simulink model "main_PETC"  (R2021a)
settings: Solver=VariableStepAuto  StartTime=0.0  StopTime=10  FixedStep=1e-4  RelTol=1e-3
InitFcn:
  | run('Parameter.m')
values from neighbouring files (symbols this model uses):
  cp = 1    [Parameter.m]
  cv = 5    [Parameter.m]
  cw = 5    [Parameter.m]
  fref = 60    [Parameter.m]
  Lc1 = 0.35e-3    (= 0.00035)    [Parameter.m]
  Lc2 = 0.35e-3    (= 0.00035)    [Parameter.m]
  Lc3 = 0.35e-3    (= 0.00035)    [Parameter.m]
  Lc4 = 0.35e-3    (= 0.00035)    [Parameter.m]
  Lt12 = 318e-6    (= 0.000318)    [Parameter.m]
  Lt23 = 1847e-6    (= 0.001847)    [Parameter.m]
  Lt34 = 318e-6    (= 0.000318)    [Parameter.m]
  Mp1 = 9.4e-5    (= 9.4e-05)    [Parameter.m]
  Mp2 = 9.4e-5    (= 9.4e-05)    [Parameter.m]
  Mp3 = 12.5e-5    (= 0.000125)    [Parameter.m]
  Mp4 = 12.5e-5    (= 0.000125)    [Parameter.m]
  Nq1 = 1.3e-3    (= 0.0013)    [Parameter.m]
  Nq2 = 1.3e-3    (= 0.0013)    [Parameter.m]
  Nq3 = 1.5e-3    (= 0.0015)    [Parameter.m]
  Nq4 = 1.5e-3    (= 0.0015)    [Parameter.m]
  Rc1 = 0.03    [Parameter.m]
  Rc2 = 0.03    [Parameter.m]
  Rc3 = 0.03    [Parameter.m]
  Rc4 = 0.03    [Parameter.m]
  Rt12 = 0.23    [Parameter.m]
  Rt23 = 0.35    [Parameter.m]
  Rt34 = 0.23    [Parameter.m]
  t2 = 1    [Parameter.m]    (also in wvpq_PETC.m)
  t3 = 10    [Parameter.m]
  t4 = 20    [Parameter.m]    (also in wvpq_PETC.m = 21)
  t5 = 35    [Parameter.m]    (also in wvpq_PETC.m = 33)
  t6 = 40    [Parameter.m]    (also in wvpq_PETC.m = 35)
  Uo = 220*sqrt(2)    [Parameter.m]
  vref = 380    [Parameter.m]
  wc = 31.4    [Parameter.m]
  wref = 2*pi*fref    (= 376.991118431)    [Parameter.m]
undefined symbols (not defined in the file or in its folder): gcbh, sps_rtmsupport
libraries: spsControlledVoltageSourceLib x12, spsAlphaBetaZerotodq0Lib x12, eeGeneralControl x8, spsThreePhaseSeriesRLCBranchLib x7, spsGroundLib x4, spsThreePhaseVIMeasurementLib x4, spsThreePhaseBreakerLib x4, spsPLL3phLib x4, spsThreePhaseSeriesRLCLoadLib x3, spspowerguiLib x1
(part 2 of 2)

== system main_PETC/controller 2/v_secondary 2 ==
  q2' : Inport
  Constant : Constant  Value=wc
  Gain1 : Gain  Gain=wc
  Gain11 : Gain  Gain=Nq2
  Gain5 : Gain  Gain=cv
  Integrator2 : Integrator  ExternalReset=rising
  Product : Product
  Step : Step  Time=t2  SampleTime=0
  Sum : Sum  Inputs=|+-
  Sum6 : Sum  Inputs=++|
  vn2 : Outport
  wires:
  [zv2] -> Gain5/1
  Sum/1 -> Gain11/1
  [q2] -> Gain1/1
  Gain11/1 -> Sum6/2
  Product/1 -> Sum/1
  q2'/1 -> Product/1
  Gain1/1 -> Sum/2
  Constant/1 -> Product/2
  Gain5/1 -> Sum6/1
  Sum6/1 -> Integrator2/1
  Step/1 -> Integrator2/2
  Integrator2/1 -> vn2/1

== system main_PETC/controller 2/w_secondary 2 ==
  Gain : Gain  Gain=cw
  Gain15 : Gain  Gain=cp
  Integrator : Integrator  ExternalReset=rising
  Step : Step  Time=t2  SampleTime=0
  Sum1 : Sum  Inputs=++|
  wn2 : Outport
  wires:
  [zp2] -> Gain15/1
  Integrator/1 -> wn2/1
  Gain15/1 -> Sum1/2
  [zw2] -> Gain/1
  Gain/1 -> Sum1/1
  Step/1 -> Integrator/2
  Sum1/1 -> Integrator/1

== system main_PETC/controller 3/(P) abc to dq2 ==
  abc : Inport  PortDimensions=3
  wt : Inport  Port=2  PortDimensions=1
  Alpha-Beta-Zero to dq0 : spsAlphaBetaZerotodq0Lib/Alpha-Beta-Zero to dq0  Alignment=90 degrees behind phase A axis
      settings: SourceProductBaseCode=PS
  abc to Alpha-Beta-Zero : Subsystem  AncestorBlock=powerlib_meascontrol/Transformations/abc to Alpha-Beta-Zero  DialogController=POWERSYS.PowerSysDialog  LoadFcn=sps_rtmsupport('LoadFcn', gcbh);  StartFcn=sps_rtmsupport('StartFcn', gcbh);  StopFcn=sps_rtmsupport('StopFcn', gcbh);  mask(abc to Alpha-Beta-Zero Transformation){}
      mask help: Perform a Clarke transformation from a three-phase (abc) signal to a alpha-beta-zero stationary reference frame.
      settings: CopyFcn=sps_rtmsupport('CopyFcn', gcbh);  DeleteFcn=sps_rtmsupport('DeleteFcn', gcbh);  UndoDeleteFcn=sps_rtmsupport('UndoDeleteFcn', gcbh);  ModelCloseFcn=sps_rtmsupport('ModelCloseFcn', gcbh);  PreSaveFcn=sps_rtmsupport('PreSaveFcn', gcbh);  PostSaveFcn=sps_rtmsupport('PostSaveFcn', gcbh);  NameChangeFcn=sps_rtmsupport('NameChangeFcn', gcbh);  PreCopyFcn=sps_rtmsupport('PreCopyFcn', gcbh);  OpenFcn=sps_rtmsupport('OpenFcn', gcbh, []);  CloseFcn=sps_rtmsupport('CloseFcn', gcbh);  PreDeleteFcn=sps_rtmsupport('PreDeleteFcn', gcbh);
      mask Help: helpview(psbhelp);
      mask Display:
      | plot([0 1], [0,1])
      | text(0.15,0.7,'abc')
      | text(0.55, 0.3,'\alpha\beta0','texmode','on')
  dq0 : Outport  VectorParamsAs1DForOutWhenUnconnected=off
  wires:
  wt/1 -> Alpha-Beta-Zero to dq0/2
  abc/1 -> abc to Alpha-Beta-Zero/1(abc)
  Alpha-Beta-Zero to dq0/1 -> dq0/1
  abc to Alpha-Beta-Zero/1(al_be_0) -> Alpha-Beta-Zero to dq0/1

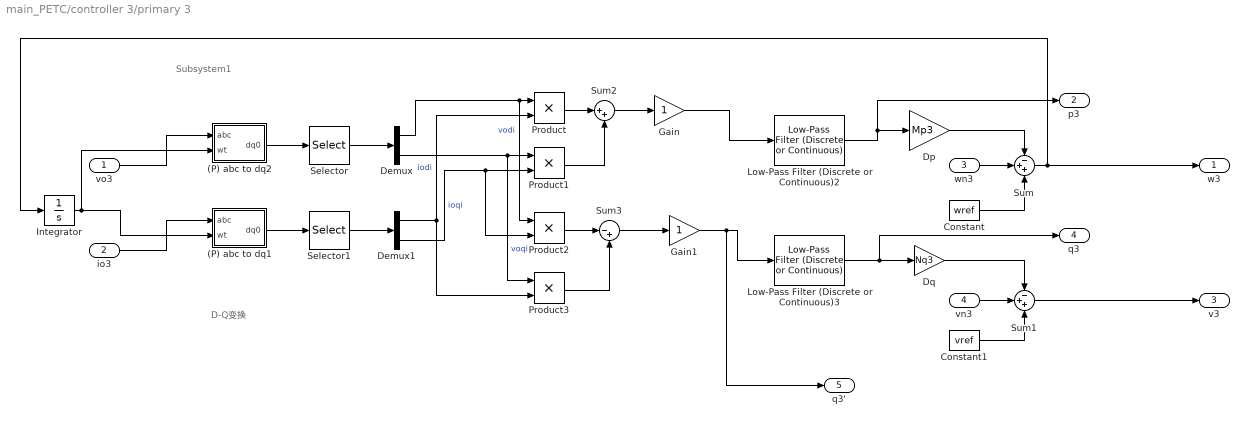
== system main_PETC/controller 3/primary 3 ==
  note: Subsystem1
  note: D-Q变换
  vo3 : Inport
  io3 : Inport  Port=2
  wn3 : Inport  Port=3
  vn3 : Inport  Port=4
  (P) abc to dq1 : Subsystem  AncestorBlock=powerlib_meascontrol/Transformations/abc to dq0  DialogController=POWERSYS.PowerSysDialog  LoadFcn=sps_rtmsupport('LoadFcn', gcbh);  StartFcn=sps_rtmsupport('StartFcn', gcbh);  StopFcn=sps_rtmsupport('StopFcn', gcbh);  mask(abc to dq0 Transformation){Alignment=90 degrees behind phase A axis}
      mask prompts: Alignment "Rotating frame alignment at wt=0:"
      mask help:
      | Perform a Park transformation from a three-phase (abc) signal to a dq0 rotating reference frame. Angular position of the rotating frame is given by input wt (rad).
      |
      | When the rotating frame alignment at wt=0 is 90 degrees behind phase A axis, a positive-sequence signal with Mag=1 & Phase=0 degrees yields the following dq values: d=1, q=0.
      mask init:
      | str=cat(2,gcb,'/Alpha-Beta-Zero to dq0');
      | if Alignment==1
      |     set_param(str,'Alignment','Aligned with phase A axis');
      | else
      |     set_param(str,'Alignment','90 degrees behind phase A axis');
      | end
      settings: CopyFcn=sps_rtmsupport('CopyFcn', gcbh);  DeleteFcn=sps_rtmsupport('DeleteFcn', gcbh);  UndoDeleteFcn=sps_rtmsupport('UndoDeleteFcn', gcbh);  ModelCloseFcn=sps_rtmsupport('ModelCloseFcn', gcbh);  PreSaveFcn=sps_rtmsupport('PreSaveFcn', gcbh);  PostSaveFcn=sps_rtmsupport('PostSaveFcn', gcbh);  NameChangeFcn=sps_rtmsupport('NameChangeFcn', gcbh);  PreCopyFcn=sps_rtmsupport('PreCopyFcn', gcbh);  OpenFcn=sps_rtmsupport('OpenFcn', gcbh, [1]);  CloseFcn=sps_rtmsupport('CloseFcn', gcbh);  PreDeleteFcn=sps_rtmsupport('PreDeleteFcn', gcbh);
      mask Help: helpview(psbhelp);
      mask TypeOptions Alignment: Aligned with phase A axis | 90 degrees behind phase A axis
      mask Display:
      | plot([0 1], [0,1])
      | port_label('input', 1, 'abc')
      | port_label('input', 2, 'wt')
      | port_label('output', 1, 'dq0')
  (P) abc to dq2 : Subsystem  AncestorBlock=powerlib_meascontrol/Transformations/abc to dq0  DialogController=POWERSYS.PowerSysDialog  LoadFcn=sps_rtmsupport('LoadFcn', gcbh);  StartFcn=sps_rtmsupport('StartFcn', gcbh);  StopFcn=sps_rtmsupport('StopFcn', gcbh);  mask(abc to dq0 Transformation){Alignment=90 degrees behind phase A axis}
      mask prompts: Alignment "Rotating frame alignment at wt=0:"
      mask help:
      | Perform a Park transformation from a three-phase (abc) signal to a dq0 rotating reference frame. Angular position of the rotating frame is given by input wt (rad).
      |
      | When the rotating frame alignment at wt=0 is 90 degrees behind phase A axis, a positive-sequence signal with Mag=1 & Phase=0 degrees yields the following dq values: d=1, q=0.
      mask init:
      | str=cat(2,gcb,'/Alpha-Beta-Zero to dq0');
      | if Alignment==1
      |     set_param(str,'Alignment','Aligned with phase A axis');
      | else
      |     set_param(str,'Alignment','90 degrees behind phase A axis');
      | end
      settings: CopyFcn=sps_rtmsupport('CopyFcn', gcbh);  DeleteFcn=sps_rtmsupport('DeleteFcn', gcbh);  UndoDeleteFcn=sps_rtmsupport('UndoDeleteFcn', gcbh);  ModelCloseFcn=sps_rtmsupport('ModelCloseFcn', gcbh);  PreSaveFcn=sps_rtmsupport('PreSaveFcn', gcbh);  PostSaveFcn=sps_rtmsupport('PostSaveFcn', gcbh);  NameChangeFcn=sps_rtmsupport('NameChangeFcn', gcbh);  PreCopyFcn=sps_rtmsupport('PreCopyFcn', gcbh);  OpenFcn=sps_rtmsupport('OpenFcn', gcbh, [1]);  CloseFcn=sps_rtmsupport('CloseFcn', gcbh);  PreDeleteFcn=sps_rtmsupport('PreDeleteFcn', gcbh);
      mask Help: helpview(psbhelp);
      mask TypeOptions Alignment: Aligned with phase A axis | 90 degrees behind phase A axis
      mask Display:
      | plot([0 1], [0,1])
      | port_label('input', 1, 'abc')
      | port_label('input', 2, 'wt')
      | port_label('output', 1, 'dq0')
  Constant : Constant  Value=wref
  Constant1 : Constant  Value=vref
  Demux : Demux  Outputs=2
  Demux1 : Demux  Outputs=2
  Dp : Gain  Gain=Mp3
  Dq : Gain  Gain=Nq3
  Gain : Gain
  Gain1 : Gain
  Integrator : Integrator
  Low-Pass Filter (Discrete or Continuous)2 : eeGeneralControl/Low-Pass Filter (Discrete or Continuous)  K=1  T=1/wc  B=inf  A=-inf  init_option=Inherited from block input  x0=0  Ts=-1
  Low-Pass Filter (Discrete or Continuous)3 : eeGeneralControl/Low-Pass Filter (Discrete or Continuous)  K=1  T=1/wc  B=inf  A=-inf  init_option=Inherited from block input  x0=0  Ts=-1
  Product{,1..3} (4 alike) : Product
  Selector : Selector  InputPortWidth=3  IndexOptions=Index vector (dialog)  Indices=[1 2]  OutputSizes=1
  Selector1 : Selector  InputPortWidth=3  IndexOptions=Index vector (dialog)  Indices=[1 2]  OutputSizes=1
  Sum : Sum  Inputs=-++
  Sum1 : Sum  Inputs=-++
  Sum2 : Sum  Inputs=|++
  Sum3 : Sum  Inputs=|-+
  w3 : Outport
  p3 : Outport  Port=2
  v3 : Outport  Port=3
  q3 : Outport  Port=4
  q3' : Outport  Port=5
  wires:
  vn3/1 -> Sum1/2
  Constant/1 -> Sum/3
  Sum1/1 -> v3/1
  Constant1/1 -> Sum1/3
  Low-Pass Filter (Discrete or Continuous)3/1 -> Dq/1, q3/1
  Sum/1 -> w3/1, Integrator/1
  Dq/1 -> Sum1/1
  wn3/1 -> Sum/2
  Dp/1 -> Sum/1
  Low-Pass Filter (Discrete or Continuous)2/1 -> Dp/1, p3/1
  Gain1/1 -> Low-Pass Filter (Discrete or Continuous)3/1, q3'/1
  Gain/1 -> Low-Pass Filter (Discrete or Continuous)2/1
  Sum3/1 -> Gain1/1
  Sum2/1 -> Gain/1
  vo3/1 -> (P) abc to dq2/1(abc)
  io3/1 -> (P) abc to dq1/1(abc)
  Product/1 -> Sum2/1
  Product1/1 -> Sum2/2
  Demux1/2 -> Product1/2, Product2/2  "ioqi"
  Product2/1 -> Sum3/1
  Product3/1 -> Sum3/2
  (P) abc to dq1/1(dq0) -> Selector1/1
  Demux1/1 -> Product3/2, Product/2  "iodi"
  (P) abc to dq2/1(dq0) -> Selector/1
  Demux/1 -> Product2/1, Product/1  "vodi"
  Integrator/1 -> (P) abc to dq1/2(wt), (P) abc to dq2/2(wt)
  Selector1/1 -> Demux1/1
  Demux/2 -> Product1/1, Product3/1  "voqi"
  Selector/1 -> Demux/1

== system main_PETC/controller 3/v_secondary 3 ==
  q3' : Inport
  Constant : Constant  Value=wc
  Gain1 : Gain  Gain=wc
  Gain11 : Gain  Gain=Nq3
  Gain5 : Gain  Gain=cv
  Integrator2 : Integrator  ExternalReset=rising
  Product : Product
  Subsystem2 : Subsystem
  Sum : Sum  Inputs=|+-
  Sum1 : Sum  Inputs=++|
  vn3 : Outport
  wires:
  [zv3] -> Gain5/1
  Gain5/1 -> Sum1/1
  Integrator2/1 -> vn3/1
  Gain11/1 -> Sum1/2
  Gain1/1 -> Sum/2
  Constant/1 -> Product/2
  q3'/1 -> Product/1
  [q3] -> Gain1/1
  Product/1 -> Sum/1
  Sum/1 -> Gain11/1
  [t] -> Integrator2/2
  Sum1/1 -> Subsystem2/1(In1)
  Subsystem2/1(Out1) -> Integrator2/1

== system main_PETC/controller 3/w_secondary 3 ==
  Gain1 : Gain  Gain=cw
  Gain15 : Gain  Gain=cp
  Integrator : Integrator  ExternalReset=rising
  Subsystem2 : Subsystem
  Sum6 : Sum  Inputs=++|
  wn3 : Outport
  wires:
  Integrator/1 -> wn3/1
  Gain15/1 -> Sum6/2
  [zw3] -> Gain1/1
  Gain1/1 -> Sum6/1
  [zp3] -> Gain15/1
  [t] -> Integrator/2
  Sum6/1 -> Subsystem2/1(In1)
  Subsystem2/1(Out1) -> Integrator/1

== system main_PETC/controller 4/(P) abc to dq2 ==
  abc : Inport  PortDimensions=3
  wt : Inport  Port=2  PortDimensions=1
  Alpha-Beta-Zero to dq0 : spsAlphaBetaZerotodq0Lib/Alpha-Beta-Zero to dq0  Alignment=90 degrees behind phase A axis
      settings: SourceProductBaseCode=PS
  abc to Alpha-Beta-Zero : Subsystem  AncestorBlock=powerlib_meascontrol/Transformations/abc to Alpha-Beta-Zero  DialogController=POWERSYS.PowerSysDialog  LoadFcn=sps_rtmsupport('LoadFcn', gcbh);  StartFcn=sps_rtmsupport('StartFcn', gcbh);  StopFcn=sps_rtmsupport('StopFcn', gcbh);  mask(abc to Alpha-Beta-Zero Transformation){}
      mask help: Perform a Clarke transformation from a three-phase (abc) signal to a alpha-beta-zero stationary reference frame.
      settings: CopyFcn=sps_rtmsupport('CopyFcn', gcbh);  DeleteFcn=sps_rtmsupport('DeleteFcn', gcbh);  UndoDeleteFcn=sps_rtmsupport('UndoDeleteFcn', gcbh);  ModelCloseFcn=sps_rtmsupport('ModelCloseFcn', gcbh);  PreSaveFcn=sps_rtmsupport('PreSaveFcn', gcbh);  PostSaveFcn=sps_rtmsupport('PostSaveFcn', gcbh);  NameChangeFcn=sps_rtmsupport('NameChangeFcn', gcbh);  PreCopyFcn=sps_rtmsupport('PreCopyFcn', gcbh);  OpenFcn=sps_rtmsupport('OpenFcn', gcbh, []);  CloseFcn=sps_rtmsupport('CloseFcn', gcbh);  PreDeleteFcn=sps_rtmsupport('PreDeleteFcn', gcbh);
      mask Help: helpview(psbhelp);
      mask Display:
      | plot([0 1], [0,1])
      | text(0.15,0.7,'abc')
      | text(0.55, 0.3,'\alpha\beta0','texmode','on')
  dq0 : Outport  VectorParamsAs1DForOutWhenUnconnected=off
  wires:
  wt/1 -> Alpha-Beta-Zero to dq0/2
  abc/1 -> abc to Alpha-Beta-Zero/1(abc)
  Alpha-Beta-Zero to dq0/1 -> dq0/1
  abc to Alpha-Beta-Zero/1(al_be_0) -> Alpha-Beta-Zero to dq0/1

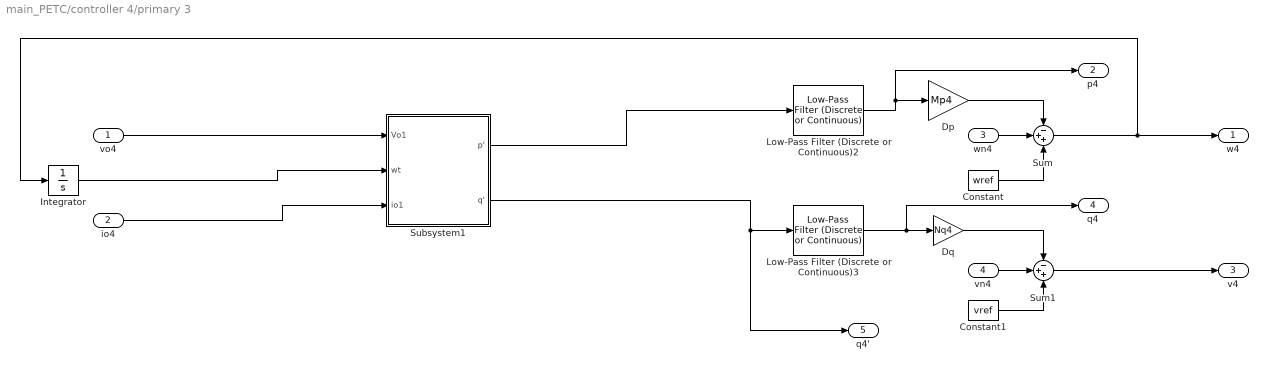
== system main_PETC/controller 4/primary 3 ==
  vo4 : Inport
  io4 : Inport  Port=2
  wn4 : Inport  Port=3
  vn4 : Inport  Port=4
  Constant : Constant  Value=wref
  Constant1 : Constant  Value=vref
  Dp : Gain  Gain=Mp4
  Dq : Gain  Gain=Nq4
  Integrator : Integrator
  Low-Pass Filter (Discrete or Continuous)2 : eeGeneralControl/Low-Pass Filter (Discrete or Continuous)  K=1  T=1/wc  B=inf  A=-inf  init_option=Inherited from block input  x0=0  Ts=-1
  Low-Pass Filter (Discrete or Continuous)3 : eeGeneralControl/Low-Pass Filter (Discrete or Continuous)  K=1  T=1/wc  B=inf  A=-inf  init_option=Inherited from block input  x0=0  Ts=-1
  Subsystem1 : Subsystem
  Sum : Sum  Inputs=-++
  Sum1 : Sum  Inputs=-++
  w4 : Outport
  p4 : Outport  Port=2
  v4 : Outport  Port=3
  q4 : Outport  Port=4
  q4' : Outport  Port=5
  wires:
  vn4/1 -> Sum1/2
  Constant/1 -> Sum/3
  Sum1/1 -> v4/1
  Constant1/1 -> Sum1/3
  Low-Pass Filter (Discrete or Continuous)3/1 -> Dq/1, q4/1
  Sum/1 -> w4/1, Integrator/1
  Dq/1 -> Sum1/1
  wn4/1 -> Sum/2
  Dp/1 -> Sum/1
  Low-Pass Filter (Discrete or Continuous)2/1 -> Dp/1, p4/1
  Subsystem1/2(q') -> Low-Pass Filter (Discrete or Continuous)3/1, q4'/1
  vo4/1 -> Subsystem1/1(Vo1)
  Integrator/1 -> Subsystem1/2(wt)
  io4/1 -> Subsystem1/3(io1)
  Subsystem1/1(p') -> Low-Pass Filter (Discrete or Continuous)2/1

== system main_PETC/controller 4/v_secondary 4 ==
  q4' : Inport
  Constant : Constant  Value=wc
  Gain1 : Gain  Gain=wc
  Gain11 : Gain  Gain=Nq4
  Gain5 : Gain  Gain=cv
  Integrator2 : Integrator  ExternalReset=rising
  Product : Product
  Step : Step  Time=t2  SampleTime=0
  Sum : Sum  Inputs=|+-
  Sum6 : Sum  Inputs=++|
  vn4 : Outport
  wires:
  [zv4] -> Gain5/1
  Integrator2/1 -> vn4/1
  Gain11/1 -> Sum6/2
  Sum6/1 -> Integrator2/1
  Gain1/1 -> Sum/2
  Constant/1 -> Product/2
  q4'/1 -> Product/1
  [q4] -> Gain1/1
  Product/1 -> Sum/1
  Sum/1 -> Gain11/1
  Step/1 -> Integrator2/2
  Gain5/1 -> Sum6/1

== system main_PETC/controller 4/w_secondary 4 ==
  Gain1 : Gain  Gain=cw
  Gain15 : Gain  Gain=cp
  Integrator : Integrator  ExternalReset=rising
  Step : Step  Time=t2  SampleTime=0
  Sum6 : Sum  Inputs=++|
  wn4 : Outport
  wires:
  Integrator/1 -> wn4/1
  Sum6/1 -> Integrator/1
  Gain15/1 -> Sum6/2
  [zw4] -> Gain1/1
  Gain1/1 -> Sum6/1
  [zp4] -> Gain15/1
  Step/1 -> Integrator/2

== system main_PETC/controller 1/(P) abc to dq2/abc to Alpha-Beta-Zero ==
  abc : Inport  PortDimensions=3
  Gain1 : Gain  Gain=sqrt(2/3)  SaturateOnIntegerOverflow=on  OutDataTypeStr=Inherit: Same as input  ParamDataTypeStr=Inherit: Same as input
  Gain3 : Gain  Gain="[ 1   -1/2   -1/2; 0   sqrt(3)/2   -sqrt(3)/2; 1/sqrt(2)  1/sqrt(2)  1/sqrt(2) ]"  Multiplication=Matrix(K*u) (u vector)  SaturateOnIntegerOverflow=on  OutDataTypeStr=Inherit: Same as input  ParamDataTypeStr=Inherit: Same as input
  al_be_0 : Outport  VectorParamsAs1DForOutWhenUnconnected=off
  wires:
  abc/1 -> Gain3/1
  Gain3/1 -> Gain1/1
  Gain1/1 -> al_be_0/1

== system main_PETC/controller 1/primary 1/(P) abc to dq1 ==
  abc : Inport  PortDimensions=3
  wt : Inport  Port=2  PortDimensions=1
  Alpha-Beta-Zero to dq0 : spsAlphaBetaZerotodq0Lib/Alpha-Beta-Zero to dq0  Alignment=90 degrees behind phase A axis
      settings: SourceProductBaseCode=PS
  abc to Alpha-Beta-Zero : Subsystem  AncestorBlock=powerlib_meascontrol/Transformations/abc to Alpha-Beta-Zero  DialogController=POWERSYS.PowerSysDialog  LoadFcn=sps_rtmsupport('LoadFcn', gcbh);  StartFcn=sps_rtmsupport('StartFcn', gcbh);  StopFcn=sps_rtmsupport('StopFcn', gcbh);  mask(abc to Alpha-Beta-Zero Transformation){}
      mask help: Perform a Clarke transformation from a three-phase (abc) signal to a alpha-beta-zero stationary reference frame.
      settings: CopyFcn=sps_rtmsupport('CopyFcn', gcbh);  DeleteFcn=sps_rtmsupport('DeleteFcn', gcbh);  UndoDeleteFcn=sps_rtmsupport('UndoDeleteFcn', gcbh);  ModelCloseFcn=sps_rtmsupport('ModelCloseFcn', gcbh);  PreSaveFcn=sps_rtmsupport('PreSaveFcn', gcbh);  PostSaveFcn=sps_rtmsupport('PostSaveFcn', gcbh);  NameChangeFcn=sps_rtmsupport('NameChangeFcn', gcbh);  PreCopyFcn=sps_rtmsupport('PreCopyFcn', gcbh);  OpenFcn=sps_rtmsupport('OpenFcn', gcbh, []);  CloseFcn=sps_rtmsupport('CloseFcn', gcbh);  PreDeleteFcn=sps_rtmsupport('PreDeleteFcn', gcbh);
      mask Help: helpview(psbhelp);
      mask Display:
      | plot([0 1], [0,1])
      | text(0.15,0.7,'abc')
      | text(0.55, 0.3,'\alpha\beta0','texmode','on')
  dq0 : Outport  VectorParamsAs1DForOutWhenUnconnected=off
  wires:
  wt/1 -> Alpha-Beta-Zero to dq0/2
  abc/1 -> abc to Alpha-Beta-Zero/1(abc)
  Alpha-Beta-Zero to dq0/1 -> dq0/1
  abc to Alpha-Beta-Zero/1(al_be_0) -> Alpha-Beta-Zero to dq0/1

== system main_PETC/controller 1/primary 1/(P) abc to dq2 ==
  abc : Inport  PortDimensions=3
  wt : Inport  Port=2  PortDimensions=1
  Alpha-Beta-Zero to dq0 : spsAlphaBetaZerotodq0Lib/Alpha-Beta-Zero to dq0  Alignment=90 degrees behind phase A axis
      settings: SourceProductBaseCode=PS
  abc to Alpha-Beta-Zero : Subsystem  AncestorBlock=powerlib_meascontrol/Transformations/abc to Alpha-Beta-Zero  DialogController=POWERSYS.PowerSysDialog  LoadFcn=sps_rtmsupport('LoadFcn', gcbh);  StartFcn=sps_rtmsupport('StartFcn', gcbh);  StopFcn=sps_rtmsupport('StopFcn', gcbh);  mask(abc to Alpha-Beta-Zero Transformation){}
      mask help: Perform a Clarke transformation from a three-phase (abc) signal to a alpha-beta-zero stationary reference frame.
      settings: CopyFcn=sps_rtmsupport('CopyFcn', gcbh);  DeleteFcn=sps_rtmsupport('DeleteFcn', gcbh);  UndoDeleteFcn=sps_rtmsupport('UndoDeleteFcn', gcbh);  ModelCloseFcn=sps_rtmsupport('ModelCloseFcn', gcbh);  PreSaveFcn=sps_rtmsupport('PreSaveFcn', gcbh);  PostSaveFcn=sps_rtmsupport('PostSaveFcn', gcbh);  NameChangeFcn=sps_rtmsupport('NameChangeFcn', gcbh);  PreCopyFcn=sps_rtmsupport('PreCopyFcn', gcbh);  OpenFcn=sps_rtmsupport('OpenFcn', gcbh, []);  CloseFcn=sps_rtmsupport('CloseFcn', gcbh);  PreDeleteFcn=sps_rtmsupport('PreDeleteFcn', gcbh);
      mask Help: helpview(psbhelp);
      mask Display:
      | plot([0 1], [0,1])
      | text(0.15,0.7,'abc')
      | text(0.55, 0.3,'\alpha\beta0','texmode','on')
  dq0 : Outport  VectorParamsAs1DForOutWhenUnconnected=off
  wires:
  wt/1 -> Alpha-Beta-Zero to dq0/2
  abc/1 -> abc to Alpha-Beta-Zero/1(abc)
  Alpha-Beta-Zero to dq0/1 -> dq0/1
  abc to Alpha-Beta-Zero/1(al_be_0) -> Alpha-Beta-Zero to dq0/1

== system main_PETC/controller 2/(P) abc to dq2/abc to Alpha-Beta-Zero ==
  abc : Inport  PortDimensions=3
  Gain1 : Gain  Gain=sqrt(2/3)  SaturateOnIntegerOverflow=on  OutDataTypeStr=Inherit: Same as input  ParamDataTypeStr=Inherit: Same as input
  Gain3 : Gain  Gain="[ 1   -1/2   -1/2; 0   sqrt(3)/2   -sqrt(3)/2; 1/sqrt(2)  1/sqrt(2)  1/sqrt(2) ]"  Multiplication=Matrix(K*u) (u vector)  SaturateOnIntegerOverflow=on  OutDataTypeStr=Inherit: Same as input  ParamDataTypeStr=Inherit: Same as input
  al_be_0 : Outport  VectorParamsAs1DForOutWhenUnconnected=off
  wires:
  abc/1 -> Gain3/1
  Gain3/1 -> Gain1/1
  Gain1/1 -> al_be_0/1

== system main_PETC/controller 2/primary 1/(P) abc to dq1 ==
  abc : Inport  PortDimensions=3
  wt : Inport  Port=2  PortDimensions=1
  Alpha-Beta-Zero to dq0 : spsAlphaBetaZerotodq0Lib/Alpha-Beta-Zero to dq0  Alignment=90 degrees behind phase A axis
      settings: SourceProductBaseCode=PS
  abc to Alpha-Beta-Zero : Subsystem  AncestorBlock=powerlib_meascontrol/Transformations/abc to Alpha-Beta-Zero  DialogController=POWERSYS.PowerSysDialog  LoadFcn=sps_rtmsupport('LoadFcn', gcbh);  StartFcn=sps_rtmsupport('StartFcn', gcbh);  StopFcn=sps_rtmsupport('StopFcn', gcbh);  mask(abc to Alpha-Beta-Zero Transformation){}
      mask help: Perform a Clarke transformation from a three-phase (abc) signal to a alpha-beta-zero stationary reference frame.
      settings: CopyFcn=sps_rtmsupport('CopyFcn', gcbh);  DeleteFcn=sps_rtmsupport('DeleteFcn', gcbh);  UndoDeleteFcn=sps_rtmsupport('UndoDeleteFcn', gcbh);  ModelCloseFcn=sps_rtmsupport('ModelCloseFcn', gcbh);  PreSaveFcn=sps_rtmsupport('PreSaveFcn', gcbh);  PostSaveFcn=sps_rtmsupport('PostSaveFcn', gcbh);  NameChangeFcn=sps_rtmsupport('NameChangeFcn', gcbh);  PreCopyFcn=sps_rtmsupport('PreCopyFcn', gcbh);  OpenFcn=sps_rtmsupport('OpenFcn', gcbh, []);  CloseFcn=sps_rtmsupport('CloseFcn', gcbh);  PreDeleteFcn=sps_rtmsupport('PreDeleteFcn', gcbh);
      mask Help: helpview(psbhelp);
      mask Display:
      | plot([0 1], [0,1])
      | text(0.15,0.7,'abc')
      | text(0.55, 0.3,'\alpha\beta0','texmode','on')
  dq0 : Outport  VectorParamsAs1DForOutWhenUnconnected=off
  wires:
  wt/1 -> Alpha-Beta-Zero to dq0/2
  abc/1 -> abc to Alpha-Beta-Zero/1(abc)
  Alpha-Beta-Zero to dq0/1 -> dq0/1
  abc to Alpha-Beta-Zero/1(al_be_0) -> Alpha-Beta-Zero to dq0/1

== system main_PETC/controller 2/primary 1/(P) abc to dq2 ==
  abc : Inport  PortDimensions=3
  wt : Inport  Port=2  PortDimensions=1
  Alpha-Beta-Zero to dq0 : spsAlphaBetaZerotodq0Lib/Alpha-Beta-Zero to dq0  Alignment=90 degrees behind phase A axis
      settings: SourceProductBaseCode=PS
  abc to Alpha-Beta-Zero : Subsystem  AncestorBlock=powerlib_meascontrol/Transformations/abc to Alpha-Beta-Zero  DialogController=POWERSYS.PowerSysDialog  LoadFcn=sps_rtmsupport('LoadFcn', gcbh);  StartFcn=sps_rtmsupport('StartFcn', gcbh);  StopFcn=sps_rtmsupport('StopFcn', gcbh);  mask(abc to Alpha-Beta-Zero Transformation){}
      mask help: Perform a Clarke transformation from a three-phase (abc) signal to a alpha-beta-zero stationary reference frame.
      settings: CopyFcn=sps_rtmsupport('CopyFcn', gcbh);  DeleteFcn=sps_rtmsupport('DeleteFcn', gcbh);  UndoDeleteFcn=sps_rtmsupport('UndoDeleteFcn', gcbh);  ModelCloseFcn=sps_rtmsupport('ModelCloseFcn', gcbh);  PreSaveFcn=sps_rtmsupport('PreSaveFcn', gcbh);  PostSaveFcn=sps_rtmsupport('PostSaveFcn', gcbh);  NameChangeFcn=sps_rtmsupport('NameChangeFcn', gcbh);  PreCopyFcn=sps_rtmsupport('PreCopyFcn', gcbh);  OpenFcn=sps_rtmsupport('OpenFcn', gcbh, []);  CloseFcn=sps_rtmsupport('CloseFcn', gcbh);  PreDeleteFcn=sps_rtmsupport('PreDeleteFcn', gcbh);
      mask Help: helpview(psbhelp);
      mask Display:
      | plot([0 1], [0,1])
      | text(0.15,0.7,'abc')
      | text(0.55, 0.3,'\alpha\beta0','texmode','on')
  dq0 : Outport  VectorParamsAs1DForOutWhenUnconnected=off
  wires:
  wt/1 -> Alpha-Beta-Zero to dq0/2
  abc/1 -> abc to Alpha-Beta-Zero/1(abc)
  Alpha-Beta-Zero to dq0/1 -> dq0/1
  abc to Alpha-Beta-Zero/1(al_be_0) -> Alpha-Beta-Zero to dq0/1

== system main_PETC/controller 3/(P) abc to dq2/abc to Alpha-Beta-Zero ==
  abc : Inport  PortDimensions=3
  Gain1 : Gain  Gain=sqrt(2/3)  SaturateOnIntegerOverflow=on  OutDataTypeStr=Inherit: Same as input  ParamDataTypeStr=Inherit: Same as input
  Gain3 : Gain  Gain="[ 1   -1/2   -1/2; 0   sqrt(3)/2   -sqrt(3)/2; 1/sqrt(2)  1/sqrt(2)  1/sqrt(2) ]"  Multiplication=Matrix(K*u) (u vector)  SaturateOnIntegerOverflow=on  OutDataTypeStr=Inherit: Same as input  ParamDataTypeStr=Inherit: Same as input
  al_be_0 : Outport  VectorParamsAs1DForOutWhenUnconnected=off
  wires:
  abc/1 -> Gain3/1
  Gain3/1 -> Gain1/1
  Gain1/1 -> al_be_0/1

== system main_PETC/controller 3/primary 3/(P) abc to dq1 ==
  abc : Inport  PortDimensions=3
  wt : Inport  Port=2  PortDimensions=1
  Alpha-Beta-Zero to dq0 : spsAlphaBetaZerotodq0Lib/Alpha-Beta-Zero to dq0  Alignment=90 degrees behind phase A axis
      settings: SourceProductBaseCode=PS
  abc to Alpha-Beta-Zero : Subsystem  AncestorBlock=powerlib_meascontrol/Transformations/abc to Alpha-Beta-Zero  DialogController=POWERSYS.PowerSysDialog  LoadFcn=sps_rtmsupport('LoadFcn', gcbh);  StartFcn=sps_rtmsupport('StartFcn', gcbh);  StopFcn=sps_rtmsupport('StopFcn', gcbh);  mask(abc to Alpha-Beta-Zero Transformation){}
      mask help: Perform a Clarke transformation from a three-phase (abc) signal to a alpha-beta-zero stationary reference frame.
      settings: CopyFcn=sps_rtmsupport('CopyFcn', gcbh);  DeleteFcn=sps_rtmsupport('DeleteFcn', gcbh);  UndoDeleteFcn=sps_rtmsupport('UndoDeleteFcn', gcbh);  ModelCloseFcn=sps_rtmsupport('ModelCloseFcn', gcbh);  PreSaveFcn=sps_rtmsupport('PreSaveFcn', gcbh);  PostSaveFcn=sps_rtmsupport('PostSaveFcn', gcbh);  NameChangeFcn=sps_rtmsupport('NameChangeFcn', gcbh);  PreCopyFcn=sps_rtmsupport('PreCopyFcn', gcbh);  OpenFcn=sps_rtmsupport('OpenFcn', gcbh, []);  CloseFcn=sps_rtmsupport('CloseFcn', gcbh);  PreDeleteFcn=sps_rtmsupport('PreDeleteFcn', gcbh);
      mask Help: helpview(psbhelp);
      mask Display:
      | plot([0 1], [0,1])
      | text(0.15,0.7,'abc')
      | text(0.55, 0.3,'\alpha\beta0','texmode','on')
  dq0 : Outport  VectorParamsAs1DForOutWhenUnconnected=off
  wires:
  wt/1 -> Alpha-Beta-Zero to dq0/2
  abc/1 -> abc to Alpha-Beta-Zero/1(abc)
  Alpha-Beta-Zero to dq0/1 -> dq0/1
  abc to Alpha-Beta-Zero/1(al_be_0) -> Alpha-Beta-Zero to dq0/1

== system main_PETC/controller 3/primary 3/(P) abc to dq2 ==
  abc : Inport  PortDimensions=3
  wt : Inport  Port=2  PortDimensions=1
  Alpha-Beta-Zero to dq0 : spsAlphaBetaZerotodq0Lib/Alpha-Beta-Zero to dq0  Alignment=90 degrees behind phase A axis
      settings: SourceProductBaseCode=PS
  abc to Alpha-Beta-Zero : Subsystem  AncestorBlock=powerlib_meascontrol/Transformations/abc to Alpha-Beta-Zero  DialogController=POWERSYS.PowerSysDialog  LoadFcn=sps_rtmsupport('LoadFcn', gcbh);  StartFcn=sps_rtmsupport('StartFcn', gcbh);  StopFcn=sps_rtmsupport('StopFcn', gcbh);  mask(abc to Alpha-Beta-Zero Transformation){}
      mask help: Perform a Clarke transformation from a three-phase (abc) signal to a alpha-beta-zero stationary reference frame.
      settings: CopyFcn=sps_rtmsupport('CopyFcn', gcbh);  DeleteFcn=sps_rtmsupport('DeleteFcn', gcbh);  UndoDeleteFcn=sps_rtmsupport('UndoDeleteFcn', gcbh);  ModelCloseFcn=sps_rtmsupport('ModelCloseFcn', gcbh);  PreSaveFcn=sps_rtmsupport('PreSaveFcn', gcbh);  PostSaveFcn=sps_rtmsupport('PostSaveFcn', gcbh);  NameChangeFcn=sps_rtmsupport('NameChangeFcn', gcbh);  PreCopyFcn=sps_rtmsupport('PreCopyFcn', gcbh);  OpenFcn=sps_rtmsupport('OpenFcn', gcbh, []);  CloseFcn=sps_rtmsupport('CloseFcn', gcbh);  PreDeleteFcn=sps_rtmsupport('PreDeleteFcn', gcbh);
      mask Help: helpview(psbhelp);
      mask Display:
      | plot([0 1], [0,1])
      | text(0.15,0.7,'abc')
      | text(0.55, 0.3,'\alpha\beta0','texmode','on')
  dq0 : Outport  VectorParamsAs1DForOutWhenUnconnected=off
  wires:
  wt/1 -> Alpha-Beta-Zero to dq0/2
  abc/1 -> abc to Alpha-Beta-Zero/1(abc)
  Alpha-Beta-Zero to dq0/1 -> dq0/1
  abc to Alpha-Beta-Zero/1(al_be_0) -> Alpha-Beta-Zero to dq0/1

== system main_PETC/controller 3/v_secondary 3/Subsystem2 ==
  In1 : Inport
  Constant : Constant  Value=0
  Switch : Switch  Criteria=u2 > Threshold
  Out1 : Outport
  wires:
  [t] -> Switch/2
  Switch/1 -> Out1/1
  Constant/1 -> Switch/3
  In1/1 -> Switch/1

== system main_PETC/controller 3/w_secondary 3/Subsystem2 ==
  In1 : Inport
  Constant : Constant  Value=0
  Switch : Switch  Criteria=u2 > Threshold
  Out1 : Outport
  wires:
  [t] -> Switch/2
  Switch/1 -> Out1/1
  Constant/1 -> Switch/3
  In1/1 -> Switch/1

== system main_PETC/controller 4/(P) abc to dq2/abc to Alpha-Beta-Zero ==
  abc : Inport  PortDimensions=3
  Gain1 : Gain  Gain=sqrt(2/3)  SaturateOnIntegerOverflow=on  OutDataTypeStr=Inherit: Same as input  ParamDataTypeStr=Inherit: Same as input
  Gain3 : Gain  Gain="[ 1   -1/2   -1/2; 0   sqrt(3)/2   -sqrt(3)/2; 1/sqrt(2)  1/sqrt(2)  1/sqrt(2) ]"  Multiplication=Matrix(K*u) (u vector)  SaturateOnIntegerOverflow=on  OutDataTypeStr=Inherit: Same as input  ParamDataTypeStr=Inherit: Same as input
  al_be_0 : Outport  VectorParamsAs1DForOutWhenUnconnected=off
  wires:
  abc/1 -> Gain3/1
  Gain3/1 -> Gain1/1
  Gain1/1 -> al_be_0/1

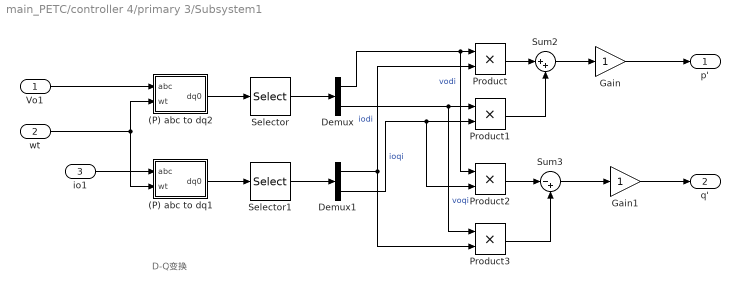
== system main_PETC/controller 4/primary 3/Subsystem1 ==
  note: D-Q变换
  Vo1 : Inport
  wt : Inport  Port=2
  io1 : Inport  Port=3
  (P) abc to dq1 : Subsystem  AncestorBlock=powerlib_meascontrol/Transformations/abc to dq0  DialogController=POWERSYS.PowerSysDialog  LoadFcn=sps_rtmsupport('LoadFcn', gcbh);  StartFcn=sps_rtmsupport('StartFcn', gcbh);  StopFcn=sps_rtmsupport('StopFcn', gcbh);  mask(abc to dq0 Transformation){Alignment=90 degrees behind phase A axis}
      mask prompts: Alignment "Rotating frame alignment at wt=0:"
      mask help:
      | Perform a Park transformation from a three-phase (abc) signal to a dq0 rotating reference frame. Angular position of the rotating frame is given by input wt (rad).
      |
      | When the rotating frame alignment at wt=0 is 90 degrees behind phase A axis, a positive-sequence signal with Mag=1 & Phase=0 degrees yields the following dq values: d=1, q=0.
      mask init:
      | str=cat(2,gcb,'/Alpha-Beta-Zero to dq0');
      | if Alignment==1
      |     set_param(str,'Alignment','Aligned with phase A axis');
      | else
      |     set_param(str,'Alignment','90 degrees behind phase A axis');
      | end
      settings: CopyFcn=sps_rtmsupport('CopyFcn', gcbh);  DeleteFcn=sps_rtmsupport('DeleteFcn', gcbh);  UndoDeleteFcn=sps_rtmsupport('UndoDeleteFcn', gcbh);  ModelCloseFcn=sps_rtmsupport('ModelCloseFcn', gcbh);  PreSaveFcn=sps_rtmsupport('PreSaveFcn', gcbh);  PostSaveFcn=sps_rtmsupport('PostSaveFcn', gcbh);  NameChangeFcn=sps_rtmsupport('NameChangeFcn', gcbh);  PreCopyFcn=sps_rtmsupport('PreCopyFcn', gcbh);  OpenFcn=sps_rtmsupport('OpenFcn', gcbh, [1]);  CloseFcn=sps_rtmsupport('CloseFcn', gcbh);  PreDeleteFcn=sps_rtmsupport('PreDeleteFcn', gcbh);
      mask Help: helpview(psbhelp);
      mask TypeOptions Alignment: Aligned with phase A axis | 90 degrees behind phase A axis
      mask Display:
      | plot([0 1], [0,1])
      | port_label('input', 1, 'abc')
      | port_label('input', 2, 'wt')
      | port_label('output', 1, 'dq0')
  (P) abc to dq2 : Subsystem  AncestorBlock=powerlib_meascontrol/Transformations/abc to dq0  DialogController=POWERSYS.PowerSysDialog  LoadFcn=sps_rtmsupport('LoadFcn', gcbh);  StartFcn=sps_rtmsupport('StartFcn', gcbh);  StopFcn=sps_rtmsupport('StopFcn', gcbh);  mask(abc to dq0 Transformation){Alignment=90 degrees behind phase A axis}
      mask prompts: Alignment "Rotating frame alignment at wt=0:"
      mask help:
      | Perform a Park transformation from a three-phase (abc) signal to a dq0 rotating reference frame. Angular position of the rotating frame is given by input wt (rad).
      |
      | When the rotating frame alignment at wt=0 is 90 degrees behind phase A axis, a positive-sequence signal with Mag=1 & Phase=0 degrees yields the following dq values: d=1, q=0.
      mask init:
      | str=cat(2,gcb,'/Alpha-Beta-Zero to dq0');
      | if Alignment==1
      |     set_param(str,'Alignment','Aligned with phase A axis');
      | else
      |     set_param(str,'Alignment','90 degrees behind phase A axis');
      | end
      settings: CopyFcn=sps_rtmsupport('CopyFcn', gcbh);  DeleteFcn=sps_rtmsupport('DeleteFcn', gcbh);  UndoDeleteFcn=sps_rtmsupport('UndoDeleteFcn', gcbh);  ModelCloseFcn=sps_rtmsupport('ModelCloseFcn', gcbh);  PreSaveFcn=sps_rtmsupport('PreSaveFcn', gcbh);  PostSaveFcn=sps_rtmsupport('PostSaveFcn', gcbh);  NameChangeFcn=sps_rtmsupport('NameChangeFcn', gcbh);  PreCopyFcn=sps_rtmsupport('PreCopyFcn', gcbh);  OpenFcn=sps_rtmsupport('OpenFcn', gcbh, [1]);  CloseFcn=sps_rtmsupport('CloseFcn', gcbh);  PreDeleteFcn=sps_rtmsupport('PreDeleteFcn', gcbh);
      mask Help: helpview(psbhelp);
      mask TypeOptions Alignment: Aligned with phase A axis | 90 degrees behind phase A axis
      mask Display:
      | plot([0 1], [0,1])
      | port_label('input', 1, 'abc')
      | port_label('input', 2, 'wt')
      | port_label('output', 1, 'dq0')
  Demux : Demux  Outputs=2
  Demux1 : Demux  Outputs=2
  Gain : Gain
  Gain1 : Gain
  Product{,1..3} (4 alike) : Product
  Selector : Selector  InputPortWidth=3  IndexOptions=Index vector (dialog)  Indices=[1 2]  OutputSizes=1
  Selector1 : Selector  InputPortWidth=3  IndexOptions=Index vector (dialog)  Indices=[1 2]  OutputSizes=1
  Sum2 : Sum  Inputs=|++
  Sum3 : Sum  Inputs=|-+
  p' : Outport
  q' : Outport  Port=2
  wires:
  Selector/1 -> Demux/1
  Demux/2 -> Product1/1, Product3/1  "voqi"
  Selector1/1 -> Demux1/1
  wt/1 -> (P) abc to dq1/2(wt), (P) abc to dq2/2(wt)
  Demux/1 -> Product2/1, Product/1  "vodi"
  (P) abc to dq2/1(dq0) -> Selector/1
  Demux1/1 -> Product3/2, Product/2  "iodi"
  (P) abc to dq1/1(dq0) -> Selector1/1
  Product3/1 -> Sum3/2
  Product2/1 -> Sum3/1
  Demux1/2 -> Product1/2, Product2/2  "ioqi"
  Product1/1 -> Sum2/2
  Product/1 -> Sum2/1
  io1/1 -> (P) abc to dq1/1(abc)
  Vo1/1 -> (P) abc to dq2/1(abc)
  Sum2/1 -> Gain/1
  Sum3/1 -> Gain1/1
  Gain1/1 -> q'/1
  Gain/1 -> p'/1

== system main_PETC/controller 1/primary 1/(P) abc to dq1/abc to Alpha-Beta-Zero ==
  abc : Inport  PortDimensions=3
  Gain1 : Gain  Gain=sqrt(2/3)  SaturateOnIntegerOverflow=on  OutDataTypeStr=Inherit: Same as input  ParamDataTypeStr=Inherit: Same as input
  Gain3 : Gain  Gain="[ 1   -1/2   -1/2; 0   sqrt(3)/2   -sqrt(3)/2; 1/sqrt(2)  1/sqrt(2)  1/sqrt(2) ]"  Multiplication=Matrix(K*u) (u vector)  SaturateOnIntegerOverflow=on  OutDataTypeStr=Inherit: Same as input  ParamDataTypeStr=Inherit: Same as input
  al_be_0 : Outport  VectorParamsAs1DForOutWhenUnconnected=off
  wires:
  abc/1 -> Gain3/1
  Gain3/1 -> Gain1/1
  Gain1/1 -> al_be_0/1

== system main_PETC/controller 1/primary 1/(P) abc to dq2/abc to Alpha-Beta-Zero ==
  abc : Inport  PortDimensions=3
  Gain1 : Gain  Gain=sqrt(2/3)  SaturateOnIntegerOverflow=on  OutDataTypeStr=Inherit: Same as input  ParamDataTypeStr=Inherit: Same as input
  Gain3 : Gain  Gain="[ 1   -1/2   -1/2; 0   sqrt(3)/2   -sqrt(3)/2; 1/sqrt(2)  1/sqrt(2)  1/sqrt(2) ]"  Multiplication=Matrix(K*u) (u vector)  SaturateOnIntegerOverflow=on  OutDataTypeStr=Inherit: Same as input  ParamDataTypeStr=Inherit: Same as input
  al_be_0 : Outport  VectorParamsAs1DForOutWhenUnconnected=off
  wires:
  abc/1 -> Gain3/1
  Gain3/1 -> Gain1/1
  Gain1/1 -> al_be_0/1

== system main_PETC/controller 2/primary 1/(P) abc to dq1/abc to Alpha-Beta-Zero ==
  abc : Inport  PortDimensions=3
  Gain1 : Gain  Gain=sqrt(2/3)  SaturateOnIntegerOverflow=on  OutDataTypeStr=Inherit: Same as input  ParamDataTypeStr=Inherit: Same as input
  Gain3 : Gain  Gain="[ 1   -1/2   -1/2; 0   sqrt(3)/2   -sqrt(3)/2; 1/sqrt(2)  1/sqrt(2)  1/sqrt(2) ]"  Multiplication=Matrix(K*u) (u vector)  SaturateOnIntegerOverflow=on  OutDataTypeStr=Inherit: Same as input  ParamDataTypeStr=Inherit: Same as input
  al_be_0 : Outport  VectorParamsAs1DForOutWhenUnconnected=off
  wires:
  abc/1 -> Gain3/1
  Gain3/1 -> Gain1/1
  Gain1/1 -> al_be_0/1

== system main_PETC/controller 2/primary 1/(P) abc to dq2/abc to Alpha-Beta-Zero ==
  abc : Inport  PortDimensions=3
  Gain1 : Gain  Gain=sqrt(2/3)  SaturateOnIntegerOverflow=on  OutDataTypeStr=Inherit: Same as input  ParamDataTypeStr=Inherit: Same as input
  Gain3 : Gain  Gain="[ 1   -1/2   -1/2; 0   sqrt(3)/2   -sqrt(3)/2; 1/sqrt(2)  1/sqrt(2)  1/sqrt(2) ]"  Multiplication=Matrix(K*u) (u vector)  SaturateOnIntegerOverflow=on  OutDataTypeStr=Inherit: Same as input  ParamDataTypeStr=Inherit: Same as input
  al_be_0 : Outport  VectorParamsAs1DForOutWhenUnconnected=off
  wires:
  abc/1 -> Gain3/1
  Gain3/1 -> Gain1/1
  Gain1/1 -> al_be_0/1

== system main_PETC/controller 3/primary 3/(P) abc to dq1/abc to Alpha-Beta-Zero ==
  abc : Inport  PortDimensions=3
  Gain1 : Gain  Gain=sqrt(2/3)  SaturateOnIntegerOverflow=on  OutDataTypeStr=Inherit: Same as input  ParamDataTypeStr=Inherit: Same as input
  Gain3 : Gain  Gain="[ 1   -1/2   -1/2; 0   sqrt(3)/2   -sqrt(3)/2; 1/sqrt(2)  1/sqrt(2)  1/sqrt(2) ]"  Multiplication=Matrix(K*u) (u vector)  SaturateOnIntegerOverflow=on  OutDataTypeStr=Inherit: Same as input  ParamDataTypeStr=Inherit: Same as input
  al_be_0 : Outport  VectorParamsAs1DForOutWhenUnconnected=off
  wires:
  abc/1 -> Gain3/1
  Gain3/1 -> Gain1/1
  Gain1/1 -> al_be_0/1

== system main_PETC/controller 3/primary 3/(P) abc to dq2/abc to Alpha-Beta-Zero ==
  abc : Inport  PortDimensions=3
  Gain1 : Gain  Gain=sqrt(2/3)  SaturateOnIntegerOverflow=on  OutDataTypeStr=Inherit: Same as input  ParamDataTypeStr=Inherit: Same as input
  Gain3 : Gain  Gain="[ 1   -1/2   -1/2; 0   sqrt(3)/2   -sqrt(3)/2; 1/sqrt(2)  1/sqrt(2)  1/sqrt(2) ]"  Multiplication=Matrix(K*u) (u vector)  SaturateOnIntegerOverflow=on  OutDataTypeStr=Inherit: Same as input  ParamDataTypeStr=Inherit: Same as input
  al_be_0 : Outport  VectorParamsAs1DForOutWhenUnconnected=off
  wires:
  abc/1 -> Gain3/1
  Gain3/1 -> Gain1/1
  Gain1/1 -> al_be_0/1

== system main_PETC/controller 4/primary 3/Subsystem1/(P) abc to dq1 ==
  abc : Inport  PortDimensions=3
  wt : Inport  Port=2  PortDimensions=1
  Alpha-Beta-Zero to dq0 : spsAlphaBetaZerotodq0Lib/Alpha-Beta-Zero to dq0  Alignment=90 degrees behind phase A axis
      settings: SourceProductBaseCode=PS
  abc to Alpha-Beta-Zero : Subsystem  AncestorBlock=powerlib_meascontrol/Transformations/abc to Alpha-Beta-Zero  DialogController=POWERSYS.PowerSysDialog  LoadFcn=sps_rtmsupport('LoadFcn', gcbh);  StartFcn=sps_rtmsupport('StartFcn', gcbh);  StopFcn=sps_rtmsupport('StopFcn', gcbh);  mask(abc to Alpha-Beta-Zero Transformation){}
      mask help: Perform a Clarke transformation from a three-phase (abc) signal to a alpha-beta-zero stationary reference frame.
      settings: CopyFcn=sps_rtmsupport('CopyFcn', gcbh);  DeleteFcn=sps_rtmsupport('DeleteFcn', gcbh);  UndoDeleteFcn=sps_rtmsupport('UndoDeleteFcn', gcbh);  ModelCloseFcn=sps_rtmsupport('ModelCloseFcn', gcbh);  PreSaveFcn=sps_rtmsupport('PreSaveFcn', gcbh);  PostSaveFcn=sps_rtmsupport('PostSaveFcn', gcbh);  NameChangeFcn=sps_rtmsupport('NameChangeFcn', gcbh);  PreCopyFcn=sps_rtmsupport('PreCopyFcn', gcbh);  OpenFcn=sps_rtmsupport('OpenFcn', gcbh, []);  CloseFcn=sps_rtmsupport('CloseFcn', gcbh);  PreDeleteFcn=sps_rtmsupport('PreDeleteFcn', gcbh);
      mask Help: helpview(psbhelp);
      mask Display:
      | plot([0 1], [0,1])
      | text(0.15,0.7,'abc')
      | text(0.55, 0.3,'\alpha\beta0','texmode','on')
  dq0 : Outport  VectorParamsAs1DForOutWhenUnconnected=off
  wires:
  wt/1 -> Alpha-Beta-Zero to dq0/2
  abc/1 -> abc to Alpha-Beta-Zero/1(abc)
  Alpha-Beta-Zero to dq0/1 -> dq0/1
  abc to Alpha-Beta-Zero/1(al_be_0) -> Alpha-Beta-Zero to dq0/1

== system main_PETC/controller 4/primary 3/Subsystem1/(P) abc to dq2 ==
  abc : Inport  PortDimensions=3
  wt : Inport  Port=2  PortDimensions=1
  Alpha-Beta-Zero to dq0 : spsAlphaBetaZerotodq0Lib/Alpha-Beta-Zero to dq0  Alignment=90 degrees behind phase A axis
      settings: SourceProductBaseCode=PS
  abc to Alpha-Beta-Zero : Subsystem  AncestorBlock=powerlib_meascontrol/Transformations/abc to Alpha-Beta-Zero  DialogController=POWERSYS.PowerSysDialog  LoadFcn=sps_rtmsupport('LoadFcn', gcbh);  StartFcn=sps_rtmsupport('StartFcn', gcbh);  StopFcn=sps_rtmsupport('StopFcn', gcbh);  mask(abc to Alpha-Beta-Zero Transformation){}
      mask help: Perform a Clarke transformation from a three-phase (abc) signal to a alpha-beta-zero stationary reference frame.
      settings: CopyFcn=sps_rtmsupport('CopyFcn', gcbh);  DeleteFcn=sps_rtmsupport('DeleteFcn', gcbh);  UndoDeleteFcn=sps_rtmsupport('UndoDeleteFcn', gcbh);  ModelCloseFcn=sps_rtmsupport('ModelCloseFcn', gcbh);  PreSaveFcn=sps_rtmsupport('PreSaveFcn', gcbh);  PostSaveFcn=sps_rtmsupport('PostSaveFcn', gcbh);  NameChangeFcn=sps_rtmsupport('NameChangeFcn', gcbh);  PreCopyFcn=sps_rtmsupport('PreCopyFcn', gcbh);  OpenFcn=sps_rtmsupport('OpenFcn', gcbh, []);  CloseFcn=sps_rtmsupport('CloseFcn', gcbh);  PreDeleteFcn=sps_rtmsupport('PreDeleteFcn', gcbh);
      mask Help: helpview(psbhelp);
      mask Display:
      | plot([0 1], [0,1])
      | text(0.15,0.7,'abc')
      | text(0.55, 0.3,'\alpha\beta0','texmode','on')
  dq0 : Outport  VectorParamsAs1DForOutWhenUnconnected=off
  wires:
  wt/1 -> Alpha-Beta-Zero to dq0/2
  abc/1 -> abc to Alpha-Beta-Zero/1(abc)
  Alpha-Beta-Zero to dq0/1 -> dq0/1
  abc to Alpha-Beta-Zero/1(al_be_0) -> Alpha-Beta-Zero to dq0/1

== system main_PETC/controller 4/primary 3/Subsystem1/(P) abc to dq1/abc to Alpha-Beta-Zero ==
  abc : Inport  PortDimensions=3
  Gain1 : Gain  Gain=sqrt(2/3)  SaturateOnIntegerOverflow=on  OutDataTypeStr=Inherit: Same as input  ParamDataTypeStr=Inherit: Same as input
  Gain3 : Gain  Gain="[ 1   -1/2   -1/2; 0   sqrt(3)/2   -sqrt(3)/2; 1/sqrt(2)  1/sqrt(2)  1/sqrt(2) ]"  Multiplication=Matrix(K*u) (u vector)  SaturateOnIntegerOverflow=on  OutDataTypeStr=Inherit: Same as input  ParamDataTypeStr=Inherit: Same as input
  al_be_0 : Outport  VectorParamsAs1DForOutWhenUnconnected=off
  wires:
  abc/1 -> Gain3/1
  Gain3/1 -> Gain1/1
  Gain1/1 -> al_be_0/1

== system main_PETC/controller 4/primary 3/Subsystem1/(P) abc to dq2/abc to Alpha-Beta-Zero ==
  abc : Inport  PortDimensions=3
  Gain1 : Gain  Gain=sqrt(2/3)  SaturateOnIntegerOverflow=on  OutDataTypeStr=Inherit: Same as input  ParamDataTypeStr=Inherit: Same as input
  Gain3 : Gain  Gain="[ 1   -1/2   -1/2; 0   sqrt(3)/2   -sqrt(3)/2; 1/sqrt(2)  1/sqrt(2)  1/sqrt(2) ]"  Multiplication=Matrix(K*u) (u vector)  SaturateOnIntegerOverflow=on  OutDataTypeStr=Inherit: Same as input  ParamDataTypeStr=Inherit: Same as input
  al_be_0 : Outport  VectorParamsAs1DForOutWhenUnconnected=off
  wires:
  abc/1 -> Gain3/1
  Gain3/1 -> Gain1/1
  Gain1/1 -> al_be_0/1

== matlab function main_PETC/line to phase1 ==
  data: u input; y output
function y = fcn(u)
xa=(2*u(1)+u(2))/3;
xc=-(2*u(2)+u(1))/3;
xb=-xa-xc;
y=[xa;xb;xc];

== matlab function main_PETC/line to phase2 ==
  data: u input; y output
function y = fcn(u)
xa=(2*u(1)+u(2))/3;
xc=-(2*u(2)+u(1))/3;
xb=-xa-xc;
y=[xa;xb;xc];

== matlab function main_PETC/line to phase3 ==
  data: u input; y output
function y = fcn(u)
xa=(2*u(1)+u(2))/3;
xc=-(2*u(2)+u(1))/3;
xb=-xa-xc;
y=[xa;xb;xc];

== matlab function main_PETC/line to phase ==
  data: u input; y output
function y = fcn(u)
xa=(2*u(1)+u(2))/3;
xc=-(2*u(2)+u(1))/3;
xb=-xa-xc;
y=[xa;xb;xc];
